simulink library "GOcontroll_Generic"  (R2018b)
settings: Solver=ode45  StartTime=0.0  StopTime=10.0  RelTol=1e-3  EnableMultiTasking=on
libraries: simulink x9, GOcontroll_Moduline_Target x9
settings Model: Creator=HANcoder  LastModifiedBy=maud
settings Model: ModifiedHistory=|
  | la_obwlf -- Thu Sep 01 12:12:55 2016 -- Version 0.33
  | 
  | 
  | 
  | 
  | 
  | 
  | la_obwlf -- Thu Sep 01 09:23:34 2016 -- Version 0.33
  | changed the version in the Base Sample Time block
  | 
  | 
  | 
  | la_obwlf -- Tue Aug 30 15:48:17 2016 -- Version 0.33
settings DataIOCC: LimitDataPoints=on  SaveFormat=Array  SignalLoggingSaveFormat=ModelDataLogs
settings OptimizationCC: ExpressionDepthLimit=2147483647  LifeSpan=inf
settings DebuggingCC: UnderspecifiedInitializationDetection=Classic  MergeDetectMultiDrivingBlocksExec=none  SolverPrmCheckMsg=warning  FcnCallInpInsideContextMsg=warning  StateNameClashWarn=warning  SFUnexpectedBacktrackingDiag=warning  SFNoUnconditionalDefaultTransitionDiag=warning  SFExecutionAtInitializationDiag=none
settings HardwareCC: ProdBitPerPointer=32  ProdBitPerSizeT=32  ProdBitPerPtrDiffT=32  ProdLargestAtomicFloat=None  ProdIntDivRoundTo=Undefined  ProdEndianess=Unspecified  ProdWordSize=32  ProdHWDeviceType=32-bit Generic
settings ModelReferenceCC: PropagateSignalLabelsOutOfModel=off
settings SFSimCC: SimUseLocalCustomCode=off
settings RTWCC: RTWUseLocalCustomCode=off
settings CodeAppCC: StateflowObjectComments=on
settings GRTTargetCC: TargetLangStandard=C89/C90 (ANSI)  GeneratePreprocessorConditionals=Disable all  CombineOutputUpdateFcns=off  GRTInterface=on
settings ConfigComp: CovMetricSettings=dw  CovHtmlReporting=on  CovSaveCumulativeToWorkspaceVar=on  CovSaveSingleToWorkspaceVar=on  CovExternalEMLEnable=off  CovSFcnEnable=off

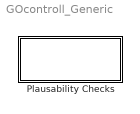
== system GOcontroll_Generic ==
  Plausability Checks : Subsystem
      settings: MoveFcn=drawLogos
      mask Display: fprintf('Plausability');

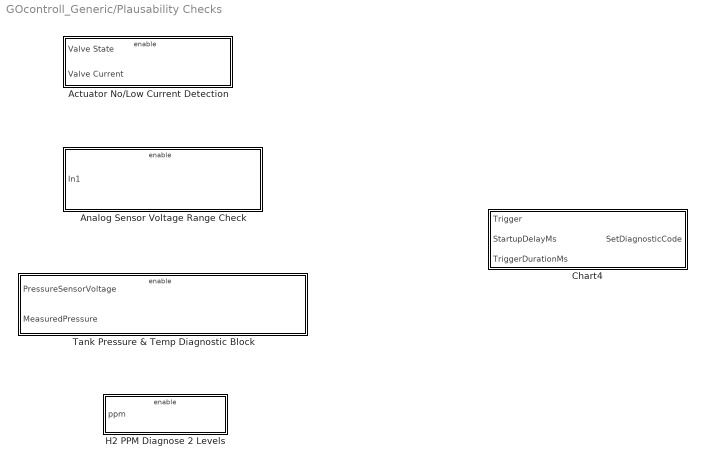
== system GOcontroll_Generic/Plausability Checks ==
  Actuator No/Low Current Detection : Subsystem  TreatAsAtomicUnit=on  mask{Signal=1}
      mask prompts: Signal "Actuator Number"
      mask Display: fprintf("Actuator no/low current detection\nActuator number: %d",Signal);
  Analog Sensor Voltage Range Check : Subsystem  mask{Signal=1, FaultCodeBase=0, TC=0, DSDelay=0, MinFaultDur=0, MinVoltage=0, MaxVoltage=0}
      mask prompts: Signal "Sensor Number"; FaultCodeBase "Fault Code Base Number"; TC "Trouble Code"; DSDelay "Diagnostics Startup Delay"; MinFaultDur "Minimum Fault Duration"; MinVoltage "Minimum Sensor Voltage"; MaxVoltage "Maximum Sensor Voltage"
      mask Display: fprintf('Analog Sensor Voltage Diagnostics\nSignal Code: %d',Signal);
  Chart4 : Stateflow chart  TreatAsAtomicUnit=on
  H2 PPM Diagnose 2 Levels : Subsystem  TreatAsAtomicUnit=on  mask{Signal=1, DSDelay=0, MinFaultDur=0, FaultBaseCode=0, TC=0}
      mask prompts: Signal "Sensor Number"; DSDelay "Diagnostic Startup Delay"; MinFaultDur "Minimal Fault Duration"; FaultBaseCode "Fault Code Base Number"; TC "Trouble Code"
      mask Display: fprintf('H2 PPM Check\nSensor Number: %d',Signal);
  Tank Pressure & Temp Diagnostic Block : Subsystem  mask{Signal=1, Cent=0, MinFaultDuration=0, DSDelay=0, MinVoltage=0, MaxVoltage=0, HighLimit1=0, HighLimit2=0, LowLimit1=0, LowLimit2=0}
      mask prompts: Cent "Fault Code Centenial value"; MinFaultDuration "Minimal Fault Duration"; DSDelay "Diagnostic Startup Delay"; MinVoltage "Minimum Sensor Voltage"; MaxVoltage "Maximum Sensor Voltage"; HighLimit1 "High Limit Level 1"; HighLimit2 "High Limit Level 2"; LowLimit1 "Low Limit Level 1"; LowLimit2 "Low Limit Level 2"
      mask help:
      | Single sensor diagnosis block for temperature and pressure sensors that come in the form:
      | 2 levels of too high and too low pressur or temp etc
      | sensor over and under voltage detection.
      mask Help:
      | Signal = number of unit it is on: Tank 1 or GHU 2 etc.
      | Fault Code Centenial Value = if a fault code is 170x11, x is the centenial value.
      | 
      | Minimal Fault duration = the time a fault needs to persist for it to trigger a diagnostic code
      | Diagnostic Startup Delay = a delay before the diagnostic system starts doing diagnostics.
      | 
      | Minimum Sensor Voltage = the lowest the voltage of a sensor is allowed to be before triggering a fault
      | Maximum Sensor Voltage = the highest the voltage of a sensor is allowed to be before triggering a fault
      | 
      | these voltage measurements are done in miliVolts
      | 
      | High Limit Level 1 = The value read by the sensor triggering the first x value is too high warning.
      | High Limit Level 2 = the value read by the sensor triggering the the warning with required action.
      | 
      | Low Limit Level 1 = The value read by the sensor triggering the first x value is too low warning.
      | Low Limit Level 2 = the value read by the sensor triggering the the warning with required action.
      | 
      | these measurements are done by the system in their unit values, celsius for temp, bar for pressure.
      mask Display: fprintf('Pressure and Temperature Sensor Diagnostics\nSignal Code: %d',Signal);

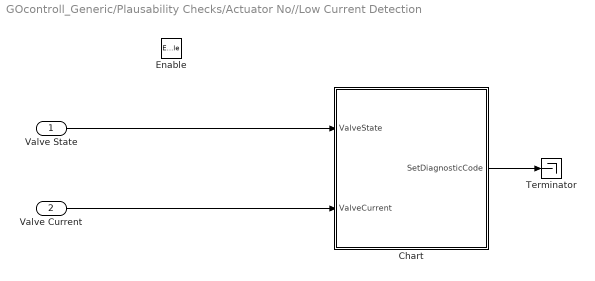
== system GOcontroll_Generic/Plausability Checks/Actuator No//Low Current Detection ==
  Valve State : Inport
  Valve Current : Inport  Port=2
  Enable : EnablePort
  Chart : Stateflow chart  TreatAsAtomicUnit=on
  Terminator : Terminator
  wires:
  Chart/1(SetDiagnosticCode) -> Terminator/1
  Valve State/1 -> Chart/1(ValveState)
  Valve Current/1 -> Chart/2(ValveCurrent)

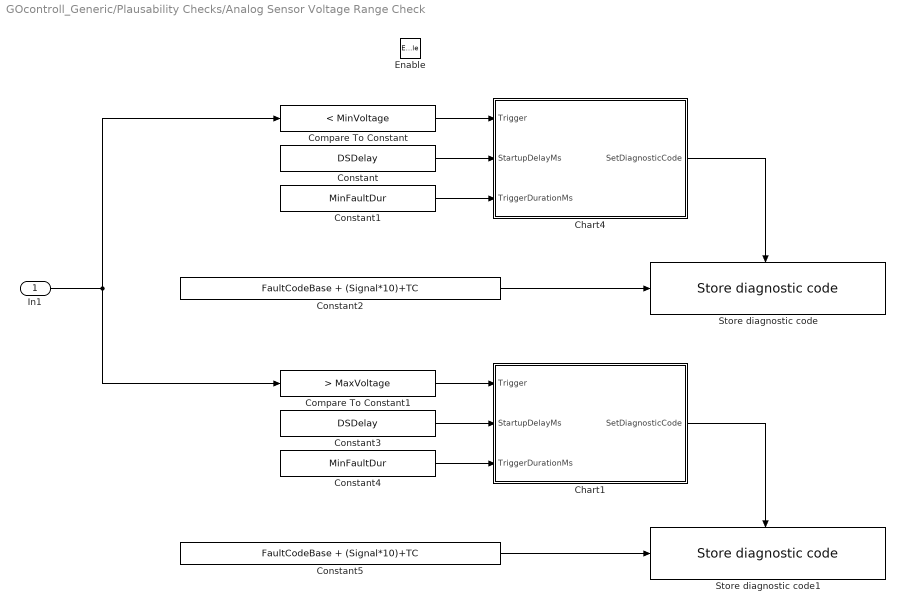
== system GOcontroll_Generic/Plausability Checks/Analog Sensor Voltage Range Check ==
  In1 : Inport
  Enable : EnablePort
  Chart1 : Stateflow chart  TreatAsAtomicUnit=on
  Chart4 : Stateflow chart  TreatAsAtomicUnit=on
  Compare To Constant : simulink/Logic and Bit Operations/Compare To Constant  relop=<  const=MinVoltage  OutDataTypeStr=boolean
  Compare To Constant1 : simulink/Logic and Bit Operations/Compare To Constant  relop=>  const=MaxVoltage  OutDataTypeStr=boolean
  Constant : Constant  Value=DSDelay  OutDataTypeStr=single
  Constant1 : Constant  Value=MinFaultDur  OutDataTypeStr=single
  Constant2 : Constant  Value=FaultCodeBase + (Signal*10)+TC  OutDataTypeStr=uint32
  Constant3 : Constant  Value=DSDelay  OutDataTypeStr=single
  Constant4 : Constant  Value=MinFaultDur  OutDataTypeStr=single
  Constant5 : Constant  Value=FaultCodeBase + (Signal*10)+TC  OutDataTypeStr=uint32
  Store diagnostic code : GOcontroll_Moduline_Target/Memory store/Diagnostic to memory/Store diagnostic code  Tag=HANcoder_GOcontroll_Moduline_IV  tsamp=-1  diagType=Warning
      settings: SourceProductName=GOcontroll Moduline
  Store diagnostic code1 : GOcontroll_Moduline_Target/Memory store/Diagnostic to memory/Store diagnostic code  Tag=HANcoder_GOcontroll_Moduline_IV  tsamp=-1  diagType=Warning
      settings: SourceProductName=GOcontroll Moduline
  wires:
  In1/1 -> Compare To Constant1/1, Compare To Constant/1
  Constant4/1 -> Chart1/3(TriggerDurationMs)
  Chart1/1(SetDiagnosticCode) -> Store diagnostic code1/Trigger
  Constant3/1 -> Chart1/2(StartupDelayMs)
  Compare To Constant1/1 -> Chart1/1(Trigger)
  Constant5/1 -> Store diagnostic code1/1
  Constant2/1 -> Store diagnostic code/1
  Compare To Constant/1 -> Chart4/1(Trigger)
  Constant/1 -> Chart4/2(StartupDelayMs)
  Chart4/1(SetDiagnosticCode) -> Store diagnostic code/Trigger
  Constant1/1 -> Chart4/3(TriggerDurationMs)

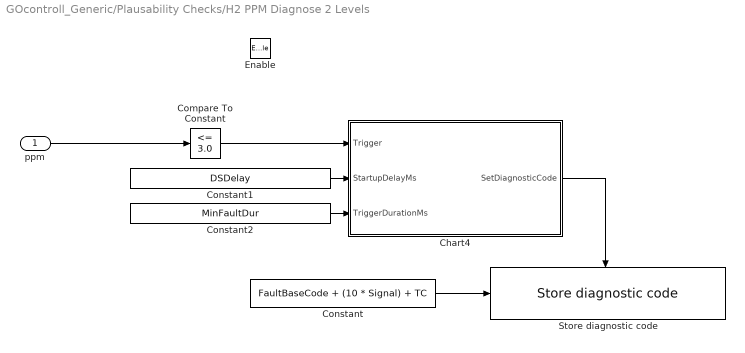
== system GOcontroll_Generic/Plausability Checks/H2 PPM Diagnose 2 Levels ==
  ppm : Inport
  Enable : EnablePort
  Chart4 : Stateflow chart  TreatAsAtomicUnit=on
  Compare To Constant : simulink/Logic and Bit Operations/Compare To Constant  relop=<=  const=3.0  OutDataTypeStr=boolean
  Constant : Constant  Value=FaultBaseCode + (10 * Signal) + TC  OutDataTypeStr=uint32
  Constant1 : Constant  Value=DSDelay  OutDataTypeStr=single
  Constant2 : Constant  Value=MinFaultDur  OutDataTypeStr=single
  Store diagnostic code : GOcontroll_Moduline_Target/Memory store/Diagnostic to memory/Store diagnostic code  Tag=HANcoder_GOcontroll_Moduline_IV  tsamp=-1  diagType=Warning
      settings: SourceProductName=GOcontroll Moduline
  wires:
  Constant2/1 -> Chart4/3(TriggerDurationMs)
  Constant1/1 -> Chart4/2(StartupDelayMs)
  Constant/1 -> Store diagnostic code/1
  Chart4/1(SetDiagnosticCode) -> Store diagnostic code/Trigger
  Compare To Constant/1 -> Chart4/1(Trigger)
  ppm/1 -> Compare To Constant/1

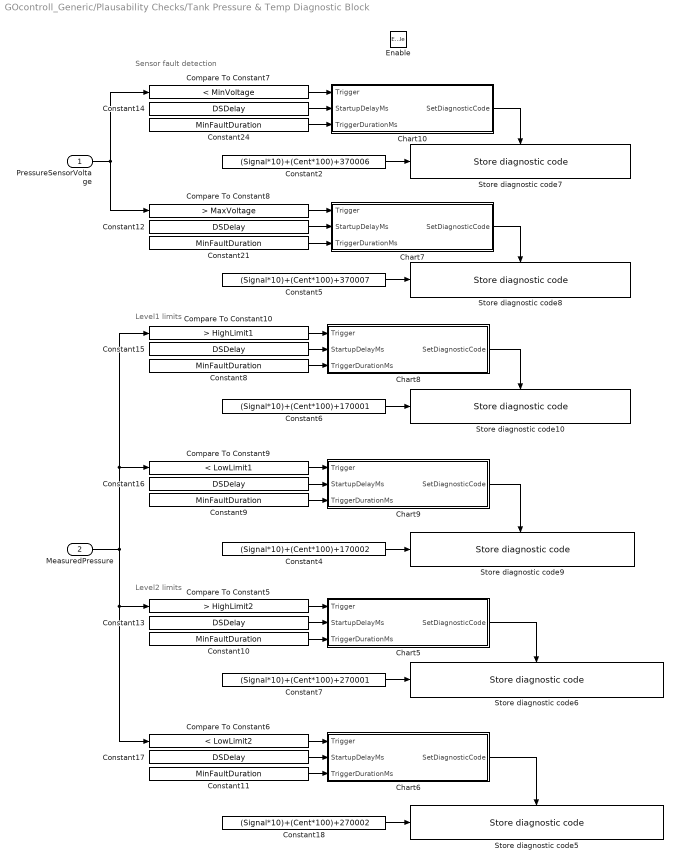
== system GOcontroll_Generic/Plausability Checks/Tank Pressure & Temp Diagnostic Block ==
  note: Level1 limits
  note: Sensor fault detection
  note: Level2 limits
  PressureSensorVoltage : Inport
  MeasuredPressure : Inport  Port=2
  Enable : EnablePort
  Chart10 : Stateflow chart  TreatAsAtomicUnit=on
  Chart5 : Stateflow chart  TreatAsAtomicUnit=on
  Chart6 : Stateflow chart  TreatAsAtomicUnit=on
  Chart7 : Stateflow chart  TreatAsAtomicUnit=on
  Chart8 : Stateflow chart  TreatAsAtomicUnit=on
  Chart9 : Stateflow chart  TreatAsAtomicUnit=on
  Compare To Constant10 : simulink/Logic and Bit Operations/Compare To Constant  relop=>  const=HighLimit1  OutDataTypeStr=boolean
  Compare To Constant5 : simulink/Logic and Bit Operations/Compare To Constant  relop=>  const=HighLimit2  OutDataTypeStr=boolean
  Compare To Constant6 : simulink/Logic and Bit Operations/Compare To Constant  relop=<  const=LowLimit2  OutDataTypeStr=boolean
  Compare To Constant7 : simulink/Logic and Bit Operations/Compare To Constant  relop=<  const=MinVoltage  OutDataTypeStr=boolean
  Compare To Constant8 : simulink/Logic and Bit Operations/Compare To Constant  relop=>  const=MaxVoltage  OutDataTypeStr=boolean
  Compare To Constant9 : simulink/Logic and Bit Operations/Compare To Constant  relop=<  const=LowLimit1  OutDataTypeStr=boolean
  Constant{8..11,21,24} (6 alike) : Constant  Value=MinFaultDuration  OutDataTypeStr=single
  Constant{12..17} (6 alike) : Constant  Value=DSDelay  OutDataTypeStr=single
  Constant18 : Constant  Value=(Signal*10)+(Cent*100)+270002  OutDataTypeStr=uint32
  Constant2 : Constant  Value=(Signal*10)+(Cent*100)+370006  OutDataTypeStr=uint32
  Constant4 : Constant  Value=(Signal*10)+(Cent*100)+170002  OutDataTypeStr=uint32
  Constant5 : Constant  Value=(Signal*10)+(Cent*100)+370007  OutDataTypeStr=uint32
  Constant6 : Constant  Value=(Signal*10)+(Cent*100)+170001  OutDataTypeStr=uint32
  Constant7 : Constant  Value=(Signal*10)+(Cent*100)+270001  OutDataTypeStr=uint32
  Store diagnostic code10 : GOcontroll_Moduline_Target/Memory store/Diagnostic to memory/Store diagnostic code  Tag=HANcoder_GOcontroll_Moduline_IV  tsamp=-1  diagType=Warning
      settings: SourceProductName=GOcontroll Moduline
  Store diagnostic code5 : GOcontroll_Moduline_Target/Memory store/Diagnostic to memory/Store diagnostic code  Tag=HANcoder_GOcontroll_Moduline_IV  tsamp=-1  diagType=Warning with action
      settings: SourceProductName=GOcontroll Moduline
  Store diagnostic code6 : GOcontroll_Moduline_Target/Memory store/Diagnostic to memory/Store diagnostic code  Tag=HANcoder_GOcontroll_Moduline_IV  tsamp=-1  diagType=Warning with action
      settings: SourceProductName=GOcontroll Moduline
  Store diagnostic code7 : GOcontroll_Moduline_Target/Memory store/Diagnostic to memory/Store diagnostic code  Tag=HANcoder_GOcontroll_Moduline_IV  tsamp=-1  diagType=Error
      settings: SourceProductName=GOcontroll Moduline
  Store diagnostic code8 : GOcontroll_Moduline_Target/Memory store/Diagnostic to memory/Store diagnostic code  Tag=HANcoder_GOcontroll_Moduline_IV  tsamp=-1  diagType=Error
      settings: SourceProductName=GOcontroll Moduline
  Store diagnostic code9 : GOcontroll_Moduline_Target/Memory store/Diagnostic to memory/Store diagnostic code  Tag=HANcoder_GOcontroll_Moduline_IV  tsamp=-1  diagType=Warning
      settings: SourceProductName=GOcontroll Moduline
  wires:
  Chart5/1(SetDiagnosticCode) -> Store diagnostic code6/Trigger
  Constant15/1 -> Chart8/2(StartupDelayMs)
  Constant7/1 -> Store diagnostic code6/1
  PressureSensorVoltage/1 -> Compare To Constant8/1, Compare To Constant7/1
  Constant9/1 -> Chart9/3(TriggerDurationMs)
  Constant6/1 -> Store diagnostic code10/1
  Constant14/1 -> Chart10/2(StartupDelayMs)
  Constant2/1 -> Store diagnostic code7/1
  Constant16/1 -> Chart9/2(StartupDelayMs)
  Constant18/1 -> Store diagnostic code5/1
  Constant21/1 -> Chart7/3(TriggerDurationMs)
  Compare To Constant8/1 -> Chart7/1(Trigger)
  MeasuredPressure/1 -> Compare To Constant5/1, Compare To Constant6/1, Compare To Constant9/1, Compare To Constant10/1
  Compare To Constant6/1 -> Chart6/1(Trigger)
  Compare To Constant10/1 -> Chart8/1(Trigger)
  Constant11/1 -> Chart6/3(TriggerDurationMs)
  Compare To Constant5/1 -> Chart5/1(Trigger)
  Chart9/1(SetDiagnosticCode) -> Store diagnostic code9/Trigger
  Chart6/1(SetDiagnosticCode) -> Store diagnostic code5/Trigger
  Constant13/1 -> Chart5/2(StartupDelayMs)
  Constant4/1 -> Store diagnostic code9/1
  Constant10/1 -> Chart5/3(TriggerDurationMs)
  Constant24/1 -> Chart10/3(TriggerDurationMs)
  Constant12/1 -> Chart7/2(StartupDelayMs)
  Constant17/1 -> Chart6/2(StartupDelayMs)
  Constant5/1 -> Store diagnostic code8/1
  Chart10/1(SetDiagnosticCode) -> Store diagnostic code7/Trigger
  Compare To Constant7/1 -> Chart10/1(Trigger)
  Chart7/1(SetDiagnosticCode) -> Store diagnostic code8/Trigger
  Chart8/1(SetDiagnosticCode) -> Store diagnostic code10/Trigger
  Compare To Constant9/1 -> Chart9/1(Trigger)
  Constant8/1 -> Chart8/3(TriggerDurationMs)

== stateflow chart GOcontroll_Generic/Plausability Checks/Tank Pressure & Temp Diagnostic Block/Chart10 ==
  state Entry
    en:SetDiagnosticCode = 0;
  state System_Running
  state Error_Triggered
  state Error_Triggered_Confirmed
    en:SetDiagnosticCode = 1;
  state Error_Code_Stored
    en:SetDiagnosticCode = 0;
  (default) -> Entry
  Entry -> System_Running : [after(StartupDelayMs,msec)]
  Error_Triggered -> System_Running [order 2] : [Trigger == 0]
  Error_Code_Stored -> System_Running
  System_Running -> Error_Triggered : [Trigger == 1]
  Error_Triggered -> Error_Triggered_Confirmed [order 1] : [after(TriggerDurationMs,msec)]
  Error_Triggered_Confirmed -> Error_Code_Stored : [after(1,sec)]
  data: Trigger input; StartupDelayMs input single; TriggerDurationMs input single; SetDiagnosticCode output uint8

== stateflow chart GOcontroll_Generic/Plausability Checks/Tank Pressure & Temp Diagnostic Block/Chart5 ==
  state Entry
    en:SetDiagnosticCode = 0;
  state System_Running
  state Error_Triggered
  state Error_Triggered_Confirmed
    en:SetDiagnosticCode = 1;
  state Error_Code_Stored
    en:SetDiagnosticCode = 0;
  (default) -> Entry
  Entry -> System_Running : [after(StartupDelayMs,msec)]
  Error_Triggered -> System_Running [order 2] : [Trigger == 0]
  Error_Code_Stored -> System_Running
  System_Running -> Error_Triggered : [Trigger == 1]
  Error_Triggered -> Error_Triggered_Confirmed [order 1] : [after(TriggerDurationMs,msec)]
  Error_Triggered_Confirmed -> Error_Code_Stored : [after(1,sec)]
  data: Trigger input; StartupDelayMs input single; TriggerDurationMs input single; SetDiagnosticCode output uint8

== stateflow chart GOcontroll_Generic/Plausability Checks/Tank Pressure & Temp Diagnostic Block/Chart6 ==
  state Entry
    en:SetDiagnosticCode = 0;
  state System_Running
  state Error_Triggered
  state Error_Triggered_Confirmed
    en:SetDiagnosticCode = 1;
  state Error_Code_Stored
    en:SetDiagnosticCode = 0;
  (default) -> Entry
  Entry -> System_Running : [after(StartupDelayMs,msec)]
  Error_Triggered -> System_Running [order 2] : [Trigger == 0]
  Error_Code_Stored -> System_Running
  System_Running -> Error_Triggered : [Trigger == 1]
  Error_Triggered -> Error_Triggered_Confirmed [order 1] : [after(TriggerDurationMs,msec)]
  Error_Triggered_Confirmed -> Error_Code_Stored : [after(1,sec)]
  data: Trigger input; StartupDelayMs input single; TriggerDurationMs input single; SetDiagnosticCode output uint8

== stateflow chart GOcontroll_Generic/Plausability Checks/Tank Pressure & Temp Diagnostic Block/Chart7 ==
  state Entry
    en:SetDiagnosticCode = 0;
  state System_Running
  state Error_Triggered
  state Error_Triggered_Confirmed
    en:SetDiagnosticCode = 1;
  state Error_Code_Stored
    en:SetDiagnosticCode = 0;
  (default) -> Entry
  Entry -> System_Running : [after(StartupDelayMs,msec)]
  Error_Triggered -> System_Running [order 2] : [Trigger == 0]
  Error_Code_Stored -> System_Running
  System_Running -> Error_Triggered : [Trigger == 1]
  Error_Triggered -> Error_Triggered_Confirmed [order 1] : [after(TriggerDurationMs,msec)]
  Error_Triggered_Confirmed -> Error_Code_Stored : [after(1,sec)]
  data: Trigger input; StartupDelayMs input single; TriggerDurationMs input single; SetDiagnosticCode output uint8

== stateflow chart GOcontroll_Generic/Plausability Checks/Tank Pressure & Temp Diagnostic Block/Chart8 ==
  state Entry
    en:SetDiagnosticCode = 0;
  state System_Running
  state Error_Triggered
  state Error_Triggered_Confirmed
    en:SetDiagnosticCode = 1;
  state Error_Code_Stored
    en:SetDiagnosticCode = 0;
  (default) -> Entry
  Entry -> System_Running : [after(StartupDelayMs,msec)]
  Error_Triggered -> System_Running [order 2] : [Trigger == 0]
  Error_Code_Stored -> System_Running
  System_Running -> Error_Triggered : [Trigger == 1]
  Error_Triggered -> Error_Triggered_Confirmed [order 1] : [after(TriggerDurationMs,msec)]
  Error_Triggered_Confirmed -> Error_Code_Stored : [after(1,sec)]
  data: Trigger input; StartupDelayMs input single; TriggerDurationMs input single; SetDiagnosticCode output uint8

== stateflow chart GOcontroll_Generic/Plausability Checks/Tank Pressure & Temp Diagnostic Block/Chart9 ==
  state Entry
    en:SetDiagnosticCode = 0;
  state System_Running
  state Error_Triggered
  state Error_Triggered_Confirmed
    en:SetDiagnosticCode = 1;
  state Error_Code_Stored
    en:SetDiagnosticCode = 0;
  (default) -> Entry
  Entry -> System_Running : [after(StartupDelayMs,msec)]
  Error_Triggered -> System_Running [order 2] : [Trigger == 0]
  Error_Code_Stored -> System_Running
  System_Running -> Error_Triggered : [Trigger == 1]
  Error_Triggered -> Error_Triggered_Confirmed [order 1] : [after(TriggerDurationMs,msec)]
  Error_Triggered_Confirmed -> Error_Code_Stored : [after(1,sec)]
  data: Trigger input; StartupDelayMs input single; TriggerDurationMs input single; SetDiagnosticCode output uint8

== stateflow chart GOcontroll_Generic/Plausability Checks/Analog Sensor Voltage Range Check/Chart1 ==
  state Entry
    en:SetDiagnosticCode = 0;
  state System_Running
  state Error_Triggered
  state Error_Triggered_Confirmed
    en:SetDiagnosticCode = 1;
  state Error_Code_Stored
    en:SetDiagnosticCode = 0;
  (default) -> Entry
  Entry -> System_Running : [after(StartupDelayMs,msec)]
  Error_Triggered -> System_Running [order 2] : [Trigger == 0]
  Error_Code_Stored -> System_Running
  System_Running -> Error_Triggered : [Trigger == 1]
  Error_Triggered -> Error_Triggered_Confirmed [order 1] : [after(TriggerDurationMs,msec)]
  Error_Triggered_Confirmed -> Error_Code_Stored : [after(1,sec)]
  data: Trigger input; StartupDelayMs input single; TriggerDurationMs input single; SetDiagnosticCode output uint8

== stateflow chart GOcontroll_Generic/Plausability Checks/Analog Sensor Voltage Range Check/Chart4 ==
  state Entry
    en:SetDiagnosticCode = 0;
  state System_Running
  state Error_Triggered
  state Error_Triggered_Confirmed
    en:SetDiagnosticCode = 1;
  state Error_Code_Stored
    en:SetDiagnosticCode = 0;
  (default) -> Entry
  Entry -> System_Running : [after(StartupDelayMs,msec)]
  Error_Triggered -> System_Running [order 2] : [Trigger == 0]
  Error_Code_Stored -> System_Running
  System_Running -> Error_Triggered : [Trigger == 1]
  Error_Triggered -> Error_Triggered_Confirmed [order 1] : [after(TriggerDurationMs,msec)]
  Error_Triggered_Confirmed -> Error_Code_Stored : [after(1,sec)]
  data: Trigger input; StartupDelayMs input single; TriggerDurationMs input single; SetDiagnosticCode output uint8

== stateflow chart GOcontroll_Generic/Plausability Checks/H2 PPM Diagnose 2 Levels/Chart4 ==
  state Entry
    en:SetDiagnosticCode = 0;
  state System_Running
  state Error_Triggered
  state Error_Triggered_Confirmed
    en:SetDiagnosticCode = 1;
  state Error_Code_Stored
    en:SetDiagnosticCode = 0;
  (default) -> Entry
  Entry -> System_Running : [after(StartupDelayMs,msec)]
  Error_Triggered -> System_Running [order 2] : [Trigger == 0]
  Error_Code_Stored -> System_Running
  System_Running -> Error_Triggered : [Trigger == 1]
  Error_Triggered -> Error_Triggered_Confirmed [order 1] : [after(TriggerDurationMs,msec)]
  Error_Triggered_Confirmed -> Error_Code_Stored : [after(1,sec)]
  data: Trigger input; StartupDelayMs input single; TriggerDurationMs input single; SetDiagnosticCode output uint8

== stateflow chart GOcontroll_Generic/Plausability Checks/Actuator No//Low Current Detection/Chart ==
  state Entry
    en:SetDiagnosticCode = 0;
  state Valve_Actuating
  state Current_Flowing
  state No_Valve_Current
    en:SetDiagnosticCode = 1;
  state Valve_Actuated
  (default) -> Entry
  Valve_Actuated -> Entry [order 2] : [ValveState==0]
  Current_Flowing -> Entry [order 3] : [ValveState==0]
  Valve_Actuating -> Entry [order 1] : [ValveState==0]
  Entry -> Valve_Actuating : [ValveState==1]
  Valve_Actuating -> Current_Flowing [order 2] : [after(100,msec)]
  Current_Flowing -> No_Valve_Current [order 2] : [after(100,msec)]
  Current_Flowing -> Valve_Actuated [order 1] : [ValveCurrent>=MinimalActuatedValveCurrent]
  Valve_Actuated -> No_Valve_Current [order 1] : [ValveCurrent<MinimalActuatedValveCurrent && ValveState==1]
  data: ValveState input; ValveCurrent input; SetDiagnosticCode output; MinimalActuatedValveCurrent parameter

== stateflow chart GOcontroll_Generic/Plausability Checks/Chart4 ==
  state Entry
    en:SetDiagnosticCode = 0;
  state System_Running
  state Error_Triggered
  state Error_Triggered_Confirmed
    en:SetDiagnosticCode = 1;
  state Error_Code_Stored
    en:SetDiagnosticCode = 0;
  (default) -> Entry
  Entry -> System_Running : [after(StartupDelayMs,msec)]
  Error_Triggered -> System_Running [order 2] : [Trigger == 0]
  Error_Code_Stored -> System_Running
  System_Running -> Error_Triggered : [Trigger == 1]
  Error_Triggered -> Error_Triggered_Confirmed [order 1] : [after(TriggerDurationMs,msec)]
  Error_Triggered_Confirmed -> Error_Code_Stored : [after(1,sec)]
  data: Trigger input; StartupDelayMs input single; TriggerDurationMs input single; SetDiagnosticCode output uint8
